simulink model "base_model_group2"  (R2022b)
settings: Solver=FixedStepAuto  StartTime=0.0  StopTime=30  FixedStep=0.01  RelTol=1e-3
values from neighbouring files (symbols this model uses):
  H_range = [-56; 38.5]    [calibration_group2.m]    (also in voltages.mat = [-56 38.5])
  HL_vrange = [min(voltages(:,2)); max(voltages(:,2))]    [calibration_group2.m]    (also in voltages.mat = [1.38451116992 3.34331548954])
  HR_vrange = [min(voltages(:,1)); max(voltages(:,1))]    [calibration_group2.m]    (also in voltages.mat = [1.95456719466 3.25506932695])
  K_range = [-137.5; 0]    [calibration_group2.m]    (also in voltages.mat = [-137.5 0])
  KL_vrange = [min(voltages(:,4)); max(voltages(:,4))]    [calibration_group2.m]    (also in voltages.mat = [0.996422290652 4.33302642896])
  KR_vrange = [min(voltages(:,3)); max(voltages(:,3))]    [calibration_group2.m]    (also in voltages.mat = [1.57034296629 4.92079941993])
undefined symbols (not defined in the file or in its folder): National_Instruments, PCIe
libraries: sldrtlib x2
settings Model: SimulationMode=external  Creator=Fox I (Daniel)  LastModifiedBy=Group 2
settings SolverCC: AlgebraicLoopSolver=TrustRegion
settings DataIOCC: ReturnWorkspaceOutputs=off
settings DebuggingCC: UnconnectedInputMsg=warning  UnconnectedOutputMsg=warning  UnconnectedLineMsg=warning  SFMachineParentedDataDiag=warning  ArithmeticOperatorsInVariantConditions=warning
settings HardwareCC: ProdBitPerLong=64  ProdHWDeviceType=Intel->x86-64 (Linux 64)
settings ModelReferenceCC: EnableRefExpFcnMdlSchedulingChecks=on
settings SFSimCC: SimUseLocalCustomCode=off  CustomCodeUndefinedFunction=UseInterfaceOnly
settings RTWCC: Description=Simulink Desktop Real-Time  SystemTargetFile=sldrt.tlc  TemplateMakefile=sldrt.tmf  RTWUseLocalCustomCode=off  RTWCompilerOptimization=on  DLArmComputeVersion=19.05
settings CodeAppCC: MaxIdLength=95
settings SimulinkDesktopRealTimeCC: TargetLibSuffix=_sldrt.a  TargetPreCompLibLocation=C:\Program Files\MATLAB\R2022b\toolbox\sldrt\lib\win64

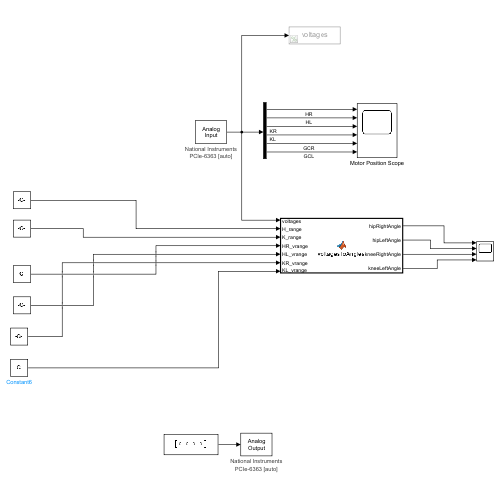
[thumbnail: Simulink's stored preview of the top-level diagram]
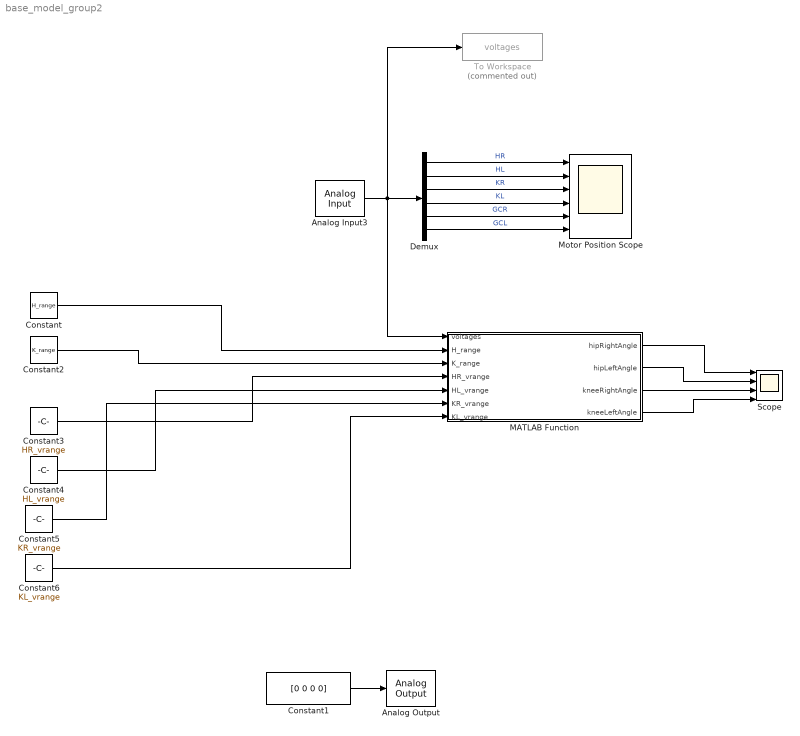
== system base_model_group2 ==
  Analog Input3 : sldrtlib/Analog Input  SampleTime=0.01  MaxMissedTicks=200  ShowMissedTicks=off  YieldWhenWaiting=off  DrvName=National_Instruments/PCIe-6363  DrvAddress=4294967295  DrvOptions=[0 0 0 0 0 0 0]  Channels=[1 2 3 4 5 6]  RangeMode=1  VoltRange=1  DataType=1
      settings: AttributesFormatString=National Instruments\nPCIe-6363 [auto]
  Analog Output : sldrtlib/Analog Output  SampleTime=0.01  MaxMissedTicks=100  ShowMissedTicks=off  YieldWhenWaiting=off  DrvName=National_Instruments/PCIe-6363  DrvAddress=4294967295  DrvOptions=[0 0 0 0 0 0 0]  Channels=[1 2 3 4]  RangeMode=1  VoltRange=1  InitialValue=0  FinalValue=0
      settings: AttributesFormatString=National Instruments\nPCIe-6363 [auto]
  Constant : Constant  Value=H_range
  Constant1 : Constant  Value=[0 0 0 0]
  Constant2 : Constant  Value=K_range
  Constant3 : Constant  Value=HR_vrange
  Constant4 : Constant  Value=HL_vrange
  Constant5 : Constant  Value=KR_vrange
  Constant6 : Constant  Value=KL_vrange
  Demux : Demux  Outputs=6
  MATLAB Function : MATLAB Function  TreatAsAtomicUnit=on
  Motor Position Scope : Scope  NumInputPorts=6
  Scope : Scope  NumInputPorts=4
  To Workspace : ToWorkspace  Commented=on  VariableName=voltages  SampleTime=-1
  wires:
  Analog Input3/1 -> MATLAB Function/1(voltages), To Workspace/1, Demux/1
  Demux/2 -> Motor Position Scope/2  "HL"
  Demux/1 -> Motor Position Scope/1  "HR"
  Demux/3 -> Motor Position Scope/3  "KR"
  Constant1/1 -> Analog Output/1
  Demux/4 -> Motor Position Scope/4  "KL"
  Demux/5 -> Motor Position Scope/5  "GCR"
  Demux/6 -> Motor Position Scope/6  "GCL"
  MATLAB Function/1(hipRightAngle) -> Scope/1
  MATLAB Function/2(hipLeftAngle) -> Scope/2
  MATLAB Function/3(kneeRightAngle) -> Scope/3
  MATLAB Function/4(kneeLeftAngle) -> Scope/4
  Constant/1 -> MATLAB Function/2(H_range)
  Constant2/1 -> MATLAB Function/3(K_range)
  Constant3/1 -> MATLAB Function/4(HR_vrange)
  Constant4/1 -> MATLAB Function/5(HL_vrange)
  Constant5/1 -> MATLAB Function/6(KR_vrange)
  Constant6/1 -> MATLAB Function/7(KL_vrange)

== matlab function base_model_group2/MATLAB Function ==
  data: voltages input; hipRightAngle output; H_range input; K_range input; HR_vrange input; HL_vrange input; KR_vrange input; KL_vrange input; hipLeftAngle output; kneeRightAngle output; kneeLeftAngle output
function [hipRightAngle, hipLeftAngle, kneeRightAngle, kneeLeftAngle] = voltagesToAngles(voltages, H_range, K_range, HR_vrange, HL_vrange, KR_vrange, KL_vrange)
    % Input validation
%     if length(voltages) ~= 4
%         error('The voltages array must contain exactly 4 elements.');
%     end

    % Extract voltage readings
    HR_voltage = voltages(1);
    HL_voltage = voltages(2);
    KR_voltage = voltages(3);
    KL_voltage = voltages(4);

    % Define ranges for hip and knee joints
    hip_min_angle = H_range(1);
    hip_max_angle = H_range(2);
    knee_min_angle = K_range(1);
    knee_max_angle = K_range(2);

    % Calculate slopes and intercepts for each joint
    HR_slope = (hip_max_angle - hip_min_angle) / (HR_vrange(2) - HR_vrange(1));
    HR_intercept = hip_min_angle - HR_slope * HR_vrange(1);
    HL_slope = (hip_max_angle - hip_min_angle) / (HL_vrange(2) - HL_vrange(1));
    HL_intercept = hip_min_angle - HL_slope * HL_vrange(1);
    KR_slope = (knee_max_angle - knee_min_angle) / (KR_vrange(2) - KR_vrange(1));
    KR_intercept = knee_min_angle - KR_slope * KR_vrange(1);
    KL_slope = (knee_max_angle - knee_min_angle) / (KL_vrange(2) - KL_vrange(1));
    KL_intercept = knee_min_angle - KL_slope * KL_vrange(1);

    % Compute the angles based on the input voltages
    hipRightAngle = HR_slope * HR_voltage + HR_intercept;
    hipLeftAngle = HL_slope * HL_voltage + HL_intercept;
    kneeRightAngle = KR_slope * KR_voltage + KR_intercept;
    kneeLeftAngle = KL_slope * KL_voltage + KL_intercept;
end
